simulink model "control_iluminacion"  (Simulink 7.5)
settings: Solver=ode45  StartTime=0.0  StopTime=200  RelTol=1e-3
libraries: fuzblock x1
settings Model: Creator=Jorge  LastModifiedBy=Jorge

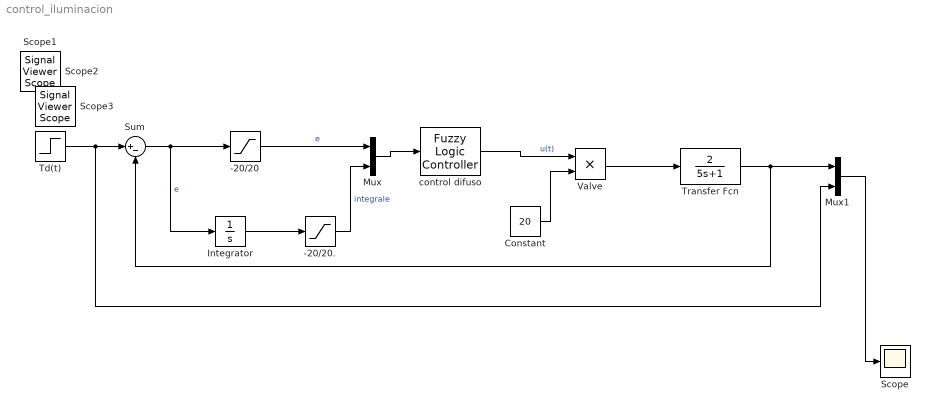
== system control_iluminacion ==
  -20/20 : Saturate  UpperLimit=20  LowerLimit=-20  OutDataType=fixdt(1, 16)  OutScaling=2^0
  -20/20. : Saturate  UpperLimit=20  LowerLimit=-20  OutDataType=fixdt(1, 16)  OutScaling=2^0
  Constant : Constant  Value=20  OutDataType=fixdt(1, 16)  OutScaling=2^0
  Integrator : Integrator
  Mux : Mux  Inputs=2
  Mux1 : Mux  Inputs=2
  Scope : Scope
      settings: YMin=0  YMax=14
  Sum : Sum  Inputs=|+-  OutDataType=fixdt(1, 16)  OutScaling=2^0
  Td(t) : Step  After=10  SampleTime=0
  Transfer Fcn : TransferFcn  Numerator=[2]  Denominator=[5 1]
  Valve : Product  OutDataType=fixdt(1, 16)  OutScaling=2^0  RndMeth=Zero
  control difuso : fuzblock/Fuzzy Logic  Controller  SystemSampleTime=-1  fis=pi_fuzzy
  Scope1 : SignalViewerScope  IOType=viewer  ZoomMode=yonly  RefreshTime=0.035000
  Scope2 : SignalViewerScope  IOType=viewer  ZoomMode=yonly  RefreshTime=0.035000
  Scope3 : SignalViewerScope  IOType=viewer  ZoomMode=xonly  RefreshTime=0.035000
      settings: YMin=-0.005  YMax=0.0005  SaveName=ScopeData2
  wires:
  Td(t)/1 -> Sum/1, Mux1/2
  Sum/1 -> -20/20/1, Integrator/1  "e"
  -20/20/1 -> Mux/1  "e"
  -20/20./1 -> Mux/2  "integrale"
  Constant/1 -> Valve/2
  Valve/1 -> Transfer Fcn/1
  Transfer Fcn/1 -> Sum/2, Mux1/1
  Mux1/1 -> Scope/1
  Mux/1 -> control difuso/1
  control difuso/1 -> Valve/1  "u(t)"
  Integrator/1 -> -20/20./1
